simulink model "TOUS_gmStateSpaceHDL_buck_convert_test1_fixpt"  (R2025a)
settings: Solver=FixedStepDiscrete  StartTime=0.0  StopTime=0.003  FixedStep=Auto  RelTol=1e-3  AbsTol=1e-3
InitFcn:
  | load('C:\Users\bensa\Desktop\PI3_FPGA_BuckConverter\sschdl\buck_convert_test1\stateSpaceParameters.mat');
model workspace (MAT data in the model file):
  NoaFutureIOMap : object (value not decoded)
undefined symbols (not defined in the file): stateSpaceParameters_1
libraries: hdlssclib x12, hdlsllib x10, library_AnalogOut x3, simulink x3
(part 2 of 2)

== system TOUS_gmStateSpaceHDL_buck_convert_test1_fixpt/FPGA/HDL Subsystem Buck-Boost/HDL Algorithm/State Update/Bias ==
  Sel : Inport  LockScale=on
  Bias : Constant  Value=single(reshape(stateSpaceParameters_1.F0d,4,4))  OutDataTypeStr=fixdt(1,32,25)  SampleTime=2.5e-08
  Data Type Conversion : DataTypeConversion  OutDataTypeStr=uint32  RndMeth=Nearest  SaturateOnIntegerOverflow=off
  Reshape : Reshape
  Selector : Selector  NumberOfDimensions=2  IndexMode=Zero-based  InputPortWidth=3  IndexOptions=Select all,Index vector (port)  Indices=[1 3]  OutputSizes=1
  Out1 : Outport  VectorParamsAs1DForOutWhenUnconnected=off
  wires:
  Selector/1 -> Reshape/1
  Bias/1 -> Selector/1
  Sel/1 -> Data Type Conversion/1
  Data Type Conversion/1 -> Selector/2
  Reshape/1 -> Out1/1

== matlab function TOUS_gmStateSpaceHDL_buck_convert_test1_fixpt/FPGA/HDL Subsystem Buck/HDL Algorithm/Mode Selection/Generate Mode Vector/Generate Mode Vector ==
  settings: fimath=fimath('RoundingMethod', 'Floor','OverflowAction', 'Wrap','ProductMode', 'FullPrecision', 'SumMode', 'FullPrecision')
  data: x input; u input; vs output; t input
function vs = compute_modes(x, u, t)

  tmp1 = ((-1.0) .* x(3));
  tmp2 = u(1);

  v1 = (tmp1 > (0.7));
  v2 = (tmp2 > (2.0));

  vs = [v1 v2];

end

== matlab function TOUS_gmStateSpaceHDL_buck_convert_test1_fixpt/FPGA/HDL Subsystem Boost/HDL Algorithm/Mode Selection/Generate Mode Vector/Generate Mode Vector ==
  data: x input; u input; vs output; t input
function vs = compute_modes(x, u, t)

  tmp1 = (((-1.0) .* x(1)) + ((-1e-06) .* x(3)) + ((-1.0) .* x(4)) + (5.0));
  tmp2 = u(1);

  v1 = (tmp1 > (0.7));
  v2 = (tmp2 > (2.0));

  vs = [v1 v2];

end

== matlab function TOUS_gmStateSpaceHDL_buck_convert_test1_fixpt/FPGA/HDL Subsystem Boost/HDL Algorithm/Mode Selection/Generate Mode Vector/Generate Mode Vector_FixPt ==
  settings: fimath=fimath('RoundingMethod', 'Floor', 'OverflowAction', 'Wrap', 'ProductMode', 'FullPrecision', 'MaxProductWordLength', 128, 'SumMode', 'FullPrecision', 'MaxSumWordLength', 128)
  data: x input; u input; vs output; t input
%auto-generated
%#codegen
function vs = compute_modes_fixpt(x, u, t)

  fm = get_fimath();
  u = fi(u, 0, 32, 29, fm);

  tmp1 = (((fi(-1.0, 1, 2, 0, fm)) .* x(1)) + ((fi(-1e-06, 1, 16, 34, fm)) .* x(3)) + ((fi(-1.0, 1, 2, 0, fm)) .* x(4)) + (fi(5.0, 0, 3, 0, fm)));
  tmp2 = fi(u(1), 0, 32, 29, fm);

  v1 = (tmp1 > (fi(0.7, 0, 16, 16, fm)));
  v2 = (tmp2 > (fi(2.0, 0, 2, 0, fm)));

  vs = [v1 v2];

end


function fm = get_fimath()
	fm = fimath('RoundingMethod', 'Floor',...
	     'OverflowAction', 'Wrap',...
	     'ProductMode','FullPrecision',...
	     'MaxProductWordLength', 128,...
	     'SumMode','FullPrecision',...
	     'MaxSumWordLength', 128);
end

== matlab function TOUS_gmStateSpaceHDL_buck_convert_test1_fixpt/FPGA/HDL Subsystem Buck-Boost/HDL Algorithm/Mode Selection/Generate Mode Vector/Generate Mode Vector ==
  data: x input; u input; vs output; t input
function vs = compute_modes(x, u, t)

  tmp1 = (x(1) + ((1e-06) .* x(3)) + ((-1.0) .* x(4)));
  tmp2 = u(1);

  v1 = (tmp1 > (0.7));
  v2 = (tmp2 > (2.0));

  vs = [v1 v2];

end

== matlab function TOUS_gmStateSpaceHDL_buck_convert_test1_fixpt/FPGA/HDL Subsystem Buck-Boost/HDL Algorithm/Mode Selection/Generate Mode Vector/Generate Mode Vector_FixPt ==
  settings: fimath=fimath('RoundingMethod', 'Floor', 'OverflowAction', 'Wrap', 'ProductMode', 'FullPrecision', 'MaxProductWordLength', 128, 'SumMode', 'FullPrecision', 'MaxSumWordLength', 128)
  data: x input; u input; vs output; t input
%auto-generated
%#codegen
function vs = compute_modes_fixpt(x, u, t)

  fm = get_fimath();
  u = fi(u, 0, 32, 29, fm);

  tmp1 = (x(1) + ((fi(1e-06, 0, 16, 35, fm)) .* x(3)) + ((fi(-1.0, 1, 2, 0, fm)) .* x(4)));
  tmp2 = fi(u(1), 0, 32, 29, fm);

  v1 = (tmp1 > (fi(0.7, 0, 16, 16, fm)));
  v2 = (tmp2 > (fi(2.0, 0, 2, 0, fm)));

  vs = [v1 v2];

end


function fm = get_fimath()
	fm = fimath('RoundingMethod', 'Floor',...
	     'OverflowAction', 'Wrap',...
	     'ProductMode','FullPrecision',...
	     'MaxProductWordLength', 128,...
	     'SumMode','FullPrecision',...
	     'MaxSumWordLength', 128);
end

== matlab function TOUS_gmStateSpaceHDL_buck_convert_test1_fixpt/FPGA/HDL Subsystem Buck/HDL Algorithm/Mode Selection/Generate Mode Vector/Generate Mode Vector_FixPt ==
  settings: fimath=fimath('RoundingMethod', 'Floor', 'OverflowAction', 'Wrap', 'ProductMode', 'FullPrecision', 'MaxProductWordLength', 128, 'SumMode', 'FullPrecision', 'MaxSumWordLength', 128)
  data: x input; u input; vs output; t input
%auto-generated
%#codegen
function vs = compute_modes_fixpt(x, u, t)

  fm = get_fimath();
  u = fi(u, 0, 32, 29, fm);

  tmp1 = ((fi(-1.0, 1, 2, 0, fm)) .* x(3));
  tmp2 = fi(u(1), 0, 32, 29, fm);

  v1 = (tmp1 > (fi(0.7, 0, 16, 16, fm)));
  v2 = (tmp2 > (fi(2.0, 0, 2, 0, fm)));

  vs = [v1 v2];

end


function fm = get_fimath()
	fm = fimath('RoundingMethod', 'Floor',...
	     'OverflowAction', 'Wrap',...
	     'ProductMode','FullPrecision',...
	     'MaxProductWordLength', 128,...
	     'SumMode','FullPrecision',...
	     'MaxSumWordLength', 128);
end
